simulink model "NonLinearPlant"  (R2020a)
settings: Solver=VariableStepAuto  StartTime=0.0  StopTime=Tsim  RelTol=1e-3
values from neighbouring files (symbols this model uses):
  Ts = 1/fs    (= 0.01)    [Model_2i2o.m]    (also in SystemIdentification.m = 0.001; exitationData.mat = 0.001; main_Simulink_Arduino_PIL_v05.m = 0.004; main_Simulink_Arduino_PIL_v05_v2.m)
  u1_step = 0.1    [SystemIdentification.m]    (also in exitationData.mat = 1)
  u1_step_time = 20    [SystemIdentification.m]    (also in exitationData.mat = 10)
  u2_step = 0.1    [SystemIdentification.m]    (also in exitationData.mat = 1)
  u2_step_time = 10    [SystemIdentification.m]    (also in exitationData.mat = 20)
  uss1 = (112.5*y_star_w - 16238*y_star_x)/1250    (= 8.740192)    [SystemIdentification.m]    (also in exitationData.mat)
  uss2 = (112.5*y_star_w + 16238*y_star_x)/1250    (= 9.259808)    [SystemIdentification.m]    (also in exitationData.mat)
libraries: slident x1
settings Model: Creator=liamw  LastModifiedBy=bezza

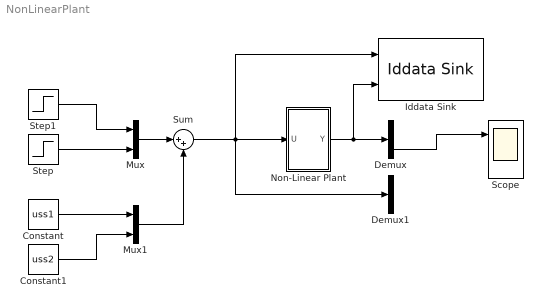
== system NonLinearPlant ==
  Constant : Constant  Value=uss1  VectorParams1D=off
  Constant1 : Constant  Value=uss2  VectorParams1D=off
  Demux : Demux  Outputs=2
  Demux1 : Demux  Outputs=2
  Iddata Sink : slident/Iddata Sink  datasetname=Data  Ts=Ts  isu=on  isy=on
      settings: SourceProductBaseCode=ID
  Mux : Mux  Inputs=2
  Mux1 : Mux  Inputs=2
  Non-Linear Plant : Subsystem
  Scope : Scope  NumInputPorts=2
  Step : Step  Time=u2_step_time  After=u2_step  SampleTime=0
  Step1 : Step  Time=u1_step_time  After=u1_step  SampleTime=0
  Sum : Sum  Inputs=|++
  wires:
  Non-Linear Plant/1(Y) -> Demux/1, Iddata Sink/2
  Mux/1 -> Sum/1
  Sum/1 -> Demux1/1, Iddata Sink/1, Non-Linear Plant/1(U)
  Step/1 -> Mux/2
  Step1/1 -> Mux/1
  Constant/1 -> Mux1/1
  Constant1/1 -> Mux1/2
  Mux1/1 -> Sum/2
  Demux/2 -> Scope/1

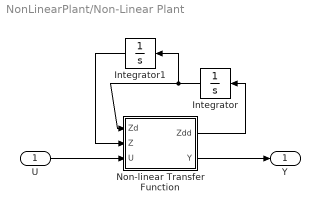
== system NonLinearPlant/Non-Linear Plant ==
  U : Inport
  Integrator : Integrator
  Integrator1 : Integrator
  Non-linear Transfer Function : MATLAB Function  TreatAsAtomicUnit=on
  Y : Outport
  wires:
  Non-linear Transfer Function/1(Zdd) -> Integrator/1
  Integrator/1 -> Integrator1/1, Non-linear Transfer Function/1(Zd)
  Integrator1/1 -> Non-linear Transfer Function/2(Z)
  Non-linear Transfer Function/2(Y) -> Y/1
  U/1 -> Non-linear Transfer Function/3(U)

== matlab function NonLinearPlant/Non-Linear Plant/Non-linear Transfer Function ==
  data: Zd input; Z input; U input; Zdd output; Y output
function [Zdd, Y]  = fcn(Zd, Z, U)
%% House keeping
Zdd=zeros(3,1);
Y = zeros(2,1);

%% System Constants
I = 0.0008;
m = 0.35;
r = 0.03;
k = 50;
ko = 200;
b = 0.09;
bo = 0.5;
h = 0.4; %height

% s = tf('s');

%% Calculate a new alpha
%x as input
x = Z(3,1);

a = atan((h/(h-x))*(sqrt(3)/3));

%a = 0.58;


%% System Matrices
M = [I 0 0;
     0 I 0;
     0 0 m];
 
B = [b 0 0;
     0 b 0;
     0 0 bo];
 
Knl = [1.5*k*r^2, -1.5*k*r^2, -k*r*cos(a);
       -1.5*k*r^2, 1.5*k*r^2, k*r*cos(a);
       -k*r*cos(a), k*r*cos(a), ko+2*k*cos(a)*cos(a)];
   
% Get the right size input   
Ua = [1 0;
      0 1;
      0 0]*U;

Zdd = (M^-1)*Ua - (M^-1)*B*Zd - (M^-1)*Knl*Z;

% Get the output we want
Y = [((Zd(1,1)+Zd(2,1))/2);   % Average of motor speeds
     Z(3,1)];                 % Tension

 
 
 
 
 
 
   
%% Transfer Functions
% Gs = ((s^2 + (M^-1)*B*s + (M^-1)*Knl)^-1)*(M^-1);
% 
% Kout = [s/2, s/2, 0;
%        0, 0, 1];
% 
% Kin = [1 0;
%        0 1;
%        0 0];
%    
% Ps = Kout*Gs*Kin;
% 
% Y = Ps*U;
